simulink model "GFM_MMC"  (R2017b)
settings: Solver=ode1  StartTime=0.0  StopTime=10.0  FixedStep=25e-6  MaxStep=200e-6  RelTol=1e-3
undefined symbols (not defined in the file): GRD00_Lg, GRD00_Rg
libraries: powerlib x15, GFM_Lib x4, VSC_Lib x1
settings Model: Creator=Frederic_Colas  LastModifiedBy=Frederic_Colas
settings DataIOCC: ReturnWorkspaceOutputs=on
settings DebuggingCC: UnconnectedInputMsg=none  UnconnectedOutputMsg=none  UnconnectedLineMsg=none  SFMachineParentedDataDiag=error
settings SFSimCC: SimUseLocalCustomCode=on
settings RTWCC: RTWUseLocalCustomCode=on

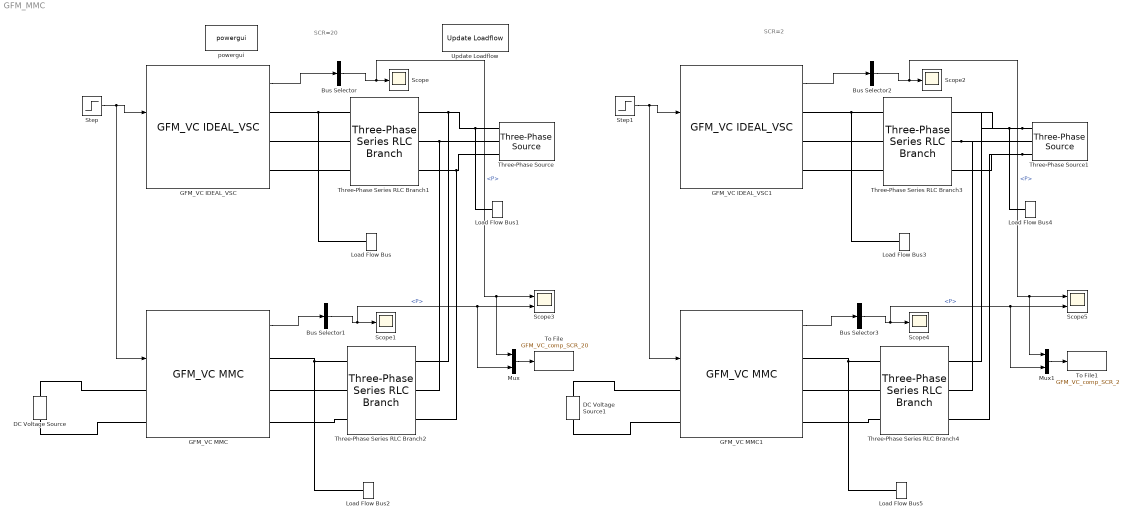
== system GFM_MMC ==
  note: SCR=20
  note: SCR=2
  Bus Selector{,1..3} (4 alike) : BusSelector  OutputSignals=P
  DC Voltage Source : powerlib/Electrical Sources/DC Voltage Source  Amplitude=640e3  Measurements=None
  DC Voltage Source1 : powerlib/Electrical Sources/DC Voltage Source  Amplitude=640e3  Measurements=None
  GFM_VC IDEAL_VSC : GFM_Lib/GFM_VC IDEAL_VSC  fn=50  Sn=1000e6  Pn=1000e6  Udcn=640e3  Output_Delay=100e-6  Un1=320e3  Un2=400e3  Rt_pu=0.005  Lt_pu=0.15+0.18/2  Lm_pu=500  Rm_pu=500  DC_Link=Perfect DC Source  H_DC=inf  H_DC_sav=40  wn_PLL=50  zeta_PLL=1  Val_Freq_Support=off  R_percent=4  dLc_pu=0  Rv=0.09  W_TVR=60  I_max_pu=1.2  wn_I_max=300  I_Max_TVI_pu=1.2  DX_DR=5  Advanced=off  gainpopup=With Inertia  wn_Inertia_Less=10  Param_Inertia=PI  H_GFo=5  zeta_GFo=1  LFpopup=PV  P0=-2.8866e-15  Q0=-9.2371e-15  V0=1  Theta0=-1.6858e-13
      settings: SourceProductName=VSC4SPS
  GFM_VC IDEAL_VSC1 : GFM_Lib/GFM_VC IDEAL_VSC  fn=50  Sn=1000e6  Pn=1000e6  Udcn=640e3  Output_Delay=100e-6  Un1=320e3  Un2=400e3  Rt_pu=0.005  Lt_pu=0.15+0.18/2  Lm_pu=500  Rm_pu=500  DC_Link=Perfect DC Source  H_DC=inf  H_DC_sav=40  wn_PLL=50  zeta_PLL=1  Val_Freq_Support=off  R_percent=4  dLc_pu=0  Rv=0.09  W_TVR=60  I_max_pu=1.2  wn_I_max=300  I_Max_TVI_pu=1.2  DX_DR=5  Advanced=off  gainpopup=With Inertia  wn_Inertia_Less=10  Param_Inertia=PI  H_GFo=5  zeta_GFo=1  LFpopup=PV  P0=-5.5511e-17  Q0=-4.4409e-16  V0=1  Theta0=-8.0309e-15
      settings: SourceProductName=VSC4SPS
  GFM_VC MMC : GFM_Lib/GFM_VC MMC  fn=50  Sn=1000e6  Pn=1000e6  Udcn=640e3  Output_Delay=100e-6  Un1=320e3  Un2=400e3  Rt_pu=0.005  Lt_pu=0.15  Lm_pu=500  Rm_pu=500  Larm_pu=0.18  Rarm_pu=0.005  nSM=0  Hc=40  DC_source=on  wn_PLL=50  zeta_PLL=1  Val_Freq_Support=off  R_percent=4  dLc_pu=0  Rv=0.09  W_TVR=60  I_max_pu=2  wn_I_max=300  I_Max_TVI_pu=2  DX_DR=5  MMC_Control_Type=Energy Based  Diff_CC_fn=200  Diff_CC_zeta=1  fn_Wtot=5  zeta_Wtot=1  fn_Wdiff=5  zeta_Wdiff=1  Advanced=on  gainpopup=With Inertia  wn_Inertia_Less=5  Param_Inertia=PI  H_GFo=5  zeta_GFo=1  LFpopup=PV  P0=-1.7764e-15  Q0=-5.3292e-15  V0=1  Theta0=-1.0428e-13
      settings: SourceProductName=VSC4SPS
  GFM_VC MMC1 : GFM_Lib/GFM_VC MMC  fn=50  Sn=1000e6  Pn=1000e6  Udcn=640e3  Output_Delay=100e-6  Un1=320e3  Un2=400e3  Rt_pu=0.005  Lt_pu=0.15  Lm_pu=500  Rm_pu=500  Larm_pu=0.18  Rarm_pu=0.005  nSM=0  Hc=40  DC_source=on  wn_PLL=50  zeta_PLL=1  Val_Freq_Support=off  R_percent=4  dLc_pu=0  Rv=0.09  W_TVR=60  I_max_pu=2  wn_I_max=300  I_Max_TVI_pu=2  DX_DR=5  MMC_Control_Type=Energy Based  Diff_CC_fn=200  Diff_CC_zeta=1  fn_Wtot=3  zeta_Wtot=1  fn_Wdiff=3  zeta_Wdiff=1  Advanced=on  gainpopup=With Inertia  wn_Inertia_Less=5  Param_Inertia=PI  H_GFo=5  zeta_GFo=1  LFpopup=PV  P0=-5.5511e-17  Q0=-1.5568e-33  V0=1  Theta0=1.6068e-15
      settings: SourceProductName=VSC4SPS
  Load Flow Bus : powerlib/Measurements/Load Flow Bus  LConnTagsString=a  Phases=single  Connectors=on one side  ID=BUS_1  Vbase=400e3  Vref=1  Vangle=0  VLF=1  VLFb=1  VLFc=1  angleLF=-1.686e-13  angleLFb=0  angleLFc=0
  Load Flow Bus1 : powerlib/Measurements/Load Flow Bus  LConnTagsString=a  Phases=single  Connectors=on one side  ID=BUS_0  Vbase=400e3  Vref=1  Vangle=0  VLF=1  VLFb=1  VLFc=1  angleLF=0  angleLFb=0  angleLFc=0
  Load Flow Bus2 : powerlib/Measurements/Load Flow Bus  LConnTagsString=a  Phases=single  Connectors=on one side  ID=BUS_3  Vbase=400e3  Vref=1  Vangle=0  VLF=1  VLFb=1  VLFc=1  angleLF=-1.043e-13  angleLFb=0  angleLFc=0
  Load Flow Bus3 : powerlib/Measurements/Load Flow Bus  LConnTagsString=a  Phases=single  Connectors=on one side  ID=BUS_5  Vbase=400e3  Vref=1  Vangle=0  VLF=1  VLFb=1  VLFc=1  angleLF=-8.031e-15  angleLFb=0  angleLFc=0
  Load Flow Bus4 : powerlib/Measurements/Load Flow Bus  LConnTagsString=a  Phases=single  Connectors=on one side  ID=BUS_4  Vbase=400e3  Vref=1  Vangle=0  VLF=1  VLFb=1  VLFc=1  angleLF=0  angleLFb=0  angleLFc=0
  Load Flow Bus5 : powerlib/Measurements/Load Flow Bus  LConnTagsString=a  Phases=single  Connectors=on one side  ID=BUS_6  Vbase=400e3  Vref=1  Vangle=0  VLF=1  VLFb=1  VLFc=1  angleLF=1.607e-15  angleLFb=0  angleLFc=0
  Mux : Mux  Inputs=2
  Mux1 : Mux  Inputs=2
  Scope{,1..2,4} (4 alike) : Scope
  Scope3 : Scope  NumInputPorts=2
  Scope5 : Scope  NumInputPorts=2
  Step : Step  Time=3  After=0.6  SampleTime=0
  Step1 : Step  Time=3  After=0.6  SampleTime=0
  Three-Phase Series RLC Branch1 : powerlib/Elements/Three-Phase Series RLC Branch  LConnTagsString=A|B|C  RConnTagsString=A|B|C  BranchType=RL  Resistance=GRD00_Rg  Inductance=GRD00_Lg  Capacitance=1e-6  Measurements=None
  Three-Phase Series RLC Branch2 : powerlib/Elements/Three-Phase Series RLC Branch  LConnTagsString=A|B|C  RConnTagsString=A|B|C  BranchType=RL  Resistance=GRD00_Rg  Inductance=GRD00_Lg  Capacitance=1e-6  Measurements=None
  Three-Phase Series RLC Branch3 : powerlib/Elements/Three-Phase Series RLC Branch  LConnTagsString=A|B|C  RConnTagsString=A|B|C  BranchType=RL  Resistance=GRD00_Rg*10  Inductance=GRD00_Lg*10  Capacitance=1e-6  Measurements=None
  Three-Phase Series RLC Branch4 : powerlib/Elements/Three-Phase Series RLC Branch  LConnTagsString=A|B|C  RConnTagsString=A|B|C  BranchType=RL  Resistance=GRD00_Rg*10  Inductance=GRD00_Lg*10  Capacitance=1e-6  Measurements=None
  Three-Phase Source : powerlib/Electrical Sources/Three-Phase Source  InternalConnection=Yg  VoltagePhases=off  Voltage=(400000)*1  PhaseAngle=0  Voltage_phases=[25e3 25e3 25e3]/sqrt(3)  PhaseAngles_phases=[0 -120 +120]  Frequency=50  NonIdealSource=off  SpecifyImpedance=on  Resistance=0.8929  Inductance=16.58e-3  ShortCircuitLevel=1e9  BaseVoltage=400e3  XRratio=10  BusType=swing  Pref=10e3  Qref=0  Prefabc=[10e3, 10e3, 10e3]  Qrefabc=[0, 0, 0]  Qmin=-inf  Qmax=inf
  Three-Phase Source1 : powerlib/Electrical Sources/Three-Phase Source  InternalConnection=Yg  VoltagePhases=off  Voltage=(400000)*1  PhaseAngle=0  Voltage_phases=[25e3 25e3 25e3]/sqrt(3)  PhaseAngles_phases=[0 -120 +120]  Frequency=50  NonIdealSource=off  SpecifyImpedance=on  Resistance=0.8929  Inductance=16.58e-3  ShortCircuitLevel=1e9  BaseVoltage=400e3  XRratio=10  BusType=swing  Pref=10e3  Qref=0  Prefabc=[10e3, 10e3, 10e3]  Qrefabc=[0, 0, 0]  Qmin=-inf  Qmax=inf
  To File : ToFile  Filename=GFM_VC_comp_SCR_20  MatrixName=power  SaveFormat=Timeseries
  To File1 : ToFile  Filename=GFM_VC_comp_SCR_2  MatrixName=power  SaveFormat=Timeseries
  Update Loadflow : VSC_Lib/Update Loadflow  ShowInLibBrowser=on
      settings: SourceProductName=VSC4SPS
  powergui : powerlib/powergui  Priority=1  SimulationMode=Discrete  SampleTime=25e-6  frequency=60  Iterations=50  frequencyindice=50  Pbase=1000000000  ErrMax=1e-6  UnitsV=kV  UnitsW=MW  buscounter=0  FunctionMessages=off  echomessages=off  EnableUseOfTLC=off  CurrentSourceSwitches=off  DisableSnubberDevices=off  DisableRonSwitches=off  DisableVfSwitches=off  DisplayEquations=off  AutomaticDiscreteSolvers=off  SolverType=Tustin/Backward Euler (TBE)  Interpol=off  ExternalGateDelay=off  methode=off  Ts=100  x0status=blocks  SPID=on  SwTol=0  HookPort=off  NonlinearTolerance=1e-4  nMaxIteration=100  ContinueOnMaxIteration=off  RestoreLinks=warning  ResistiveCurrentMeasurement=off  Frange=[0:2:500]  Ylog=off  Xlog=on  ShowGrid=off  save=off  variable=ZData  structure=0  ZoomFFT=off  StartTime=0.0  cycles=1  DisplayStyle=1  fundamental=60  FreqAxis=off  MaxFrequency=1000  frequencyindicesteady=1  RmsSteady=1  display=off
  wires:
  GFM_VC IDEAL_VSC/1 -> Bus Selector/1
  Bus Selector/1 -> Mux/1, Scope3/1, Scope/1  "<P>"
  Step/1 -> GFM_VC MMC/2, GFM_VC IDEAL_VSC/2
  Bus Selector1/1 -> Mux/2, Scope3/2, Scope1/1  "<P>"
  GFM_VC MMC/1 -> Bus Selector1/1
  Mux/1 -> To File/1
  Bus Selector2/1 -> Mux1/1, Scope5/1, Scope2/1  "<P>"
  GFM_VC MMC1/1 -> Bus Selector3/1
  Bus Selector3/1 -> Mux1/2, Scope5/2, Scope4/1  "<P>"
  Step1/1 -> GFM_VC MMC1/2, GFM_VC IDEAL_VSC1/2
  Mux1/1 -> To File1/1
  GFM_VC IDEAL_VSC1/1 -> Bus Selector2/1
  connections:
  Three-Phase Series RLC Branch1/LConn1 -- GFM_VC IDEAL_VSC/RConn1 -- Load Flow Bus/LConn1
  GFM_VC IDEAL_VSC/RConn2 -- Three-Phase Series RLC Branch1/LConn2
  GFM_VC IDEAL_VSC/RConn3 -- Three-Phase Series RLC Branch1/LConn3
  Three-Phase Series RLC Branch1/RConn1 -- Three-Phase Series RLC Branch2/RConn1 -- Load Flow Bus1/LConn1 -- Three-Phase Source/RConn1
  Three-Phase Source/RConn2 -- Three-Phase Series RLC Branch2/RConn2 -- Three-Phase Series RLC Branch1/RConn2
  Three-Phase Series RLC Branch1/RConn3 -- Three-Phase Series RLC Branch2/RConn3 -- Three-Phase Source/RConn3
  Load Flow Bus2/LConn1 -- Three-Phase Series RLC Branch2/LConn1 -- GFM_VC MMC/RConn1
  GFM_VC MMC/RConn2 -- Three-Phase Series RLC Branch2/LConn2
  GFM_VC MMC/RConn3 -- Three-Phase Series RLC Branch2/LConn3
  GFM_VC MMC/LConn1 -- DC Voltage Source/RConn1
  GFM_VC MMC/LConn2 -- DC Voltage Source/LConn1
  Three-Phase Series RLC Branch3/RConn2 -- Three-Phase Source1/RConn2 -- Three-Phase Series RLC Branch4/RConn2
  GFM_VC MMC1/RConn1 -- Load Flow Bus5/LConn1 -- Three-Phase Series RLC Branch4/LConn1
  Three-Phase Source1/RConn1 -- Three-Phase Series RLC Branch3/RConn1 -- Three-Phase Series RLC Branch4/RConn1 -- Load Flow Bus4/LConn1
  Load Flow Bus3/LConn1 -- Three-Phase Series RLC Branch3/LConn1 -- GFM_VC IDEAL_VSC1/RConn1
  Three-Phase Source1/RConn3 -- Three-Phase Series RLC Branch3/RConn3 -- Three-Phase Series RLC Branch4/RConn3
  GFM_VC MMC1/RConn2 -- Three-Phase Series RLC Branch4/LConn2
  GFM_VC IDEAL_VSC1/RConn3 -- Three-Phase Series RLC Branch3/LConn3
  GFM_VC IDEAL_VSC1/RConn2 -- Three-Phase Series RLC Branch3/LConn2
  GFM_VC MMC1/LConn2 -- DC Voltage Source1/LConn1
  GFM_VC MMC1/LConn1 -- DC Voltage Source1/RConn1
  GFM_VC MMC1/RConn3 -- Three-Phase Series RLC Branch4/LConn3
